simulink model "project1"  (R2014a)
settings: Solver=ode45  StartTime=0.0  StopTime=1.5  FixedStep=0.0015
libraries: powerlib x9, powerlib_meascontrol x1
settings Model: Creator=yusuf  LastModifiedBy=yusuf

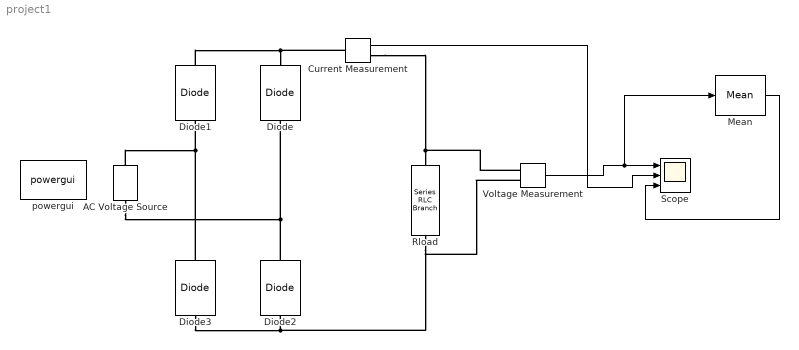
== system project1 ==
  AC Voltage Source : powerlib/Electrical Sources/AC Voltage Source  Amplitude=230.9  Phase=0  Frequency=50  SampleTime=0  Measurements=None
  Current Measurement : powerlib/Measurements/Current Measurement  PhasorSimulation=off  OutputType=Complex  PSBequivalent=0
  Diode{,1..3} (4 alike) : powerlib/Power Electronics/Diode  Ron=0.001  Lon=0  Vf=0.8  IC=0  UseSnubber=off  Rs=500  Cs=250e-9  Measurements=off
  Mean : powerlib_meascontrol/Measurements/Mean  Freq=60  Vinit=0  Ts=0
  Rload : powerlib/Elements/Series RLC Branch  LConnTagsString=__new0  RConnTagsString=__new0  BranchType=RL  Resistance=25  Inductance=1  SetiL0=off  InitialCurrent=0  Capacitance=1e-6  Setx0=off  InitialVoltage=0  Measurements=None
  Scope : Scope  NumInputPorts=3
      settings: TickLabels=on  ShowLegends=on  TimeRange=0.1  YMin=0~-5~-5  YMax=250~5~5
  Voltage Measurement : powerlib/Measurements/Voltage Measurement  PhasorSimulation=off  OutputType=Complex  PSBequivalent=0
  powergui : powerlib/powergui  Priority=1  SimulationMode=Discrete  SolverType=Tustin  SampleTime=1e-6  frequency=60  SPID=off  DisableSnubberDevices=off  DisableRonSwitches=off  DisableVfSwitches=off  SwTol=0  Interpol=off  DisplayEquations=off  Ts=0  methode=off  frequencyindice=50  Pbase=100e6  ErrMax=1e-4  Iterations=50  UnitsV=kV  UnitsW=MW  FunctionMessages=off  echomessages=off  HookPort=off  EnableUseOfTLC=off  x0status=blocks  RestoreLinks=warning  ResistiveCurrentMeasurement=off  Frange=[0:2:500]  Ylog=off  Xlog=on  ShowGrid=off  save=off  variable=ZData  structure=0  ZoomFFT=off  StartTime=0.0  cycles=1  DisplayStyle=1  fundamental=60  FreqAxis=off  MaxFrequency=1000  frequencyindicesteady=1  RmsSteady=1  display=off
  wires:
  Current Measurement/1 -> Scope/2
  Voltage Measurement/1 -> Mean/1, Scope/1
  Mean/1 -> Scope/3
  connections:
  Diode1/RConn1 -- Current Measurement/LConn1 -- Diode/RConn1
  Diode3/RConn1 -- AC Voltage Source/RConn1 -- Diode1/LConn1
  Diode2/RConn1 -- AC Voltage Source/LConn1 -- Diode/LConn1
  Diode3/LConn1 -- Rload/LConn1 -- Voltage Measurement/LConn2 -- Diode2/LConn1
  Voltage Measurement/LConn1 -- Current Measurement/RConn1 -- Rload/RConn1
